simulink model "model_downsampling"  (R2021b)
settings: Solver=VariableStepAuto  StartTime=0.0  StopTime=3  RelTol=1e-3
values from neighbouring files (symbols this model uses):
  dowsampling_factor = 32    [init_model.m]
  fsample = 100e3    (= 100000)    [init_model.m]
  m1 = m1_th    [init_model.m]
  m2 = m2_th    [init_model.m]
  taps = fir1(floor(n),fpass/fsample)    [init_model.m]
  taps1 = fir1(floor(n1),fpass1/fsample)    [init_model.m]
libraries: simulink x3
settings Model: Creator=pablo  LastModifiedBy=pablo
settings SolverCC: AutoInsertRateTranBlk=on
settings DebuggingCC: SingleTaskRateTransMsg=error

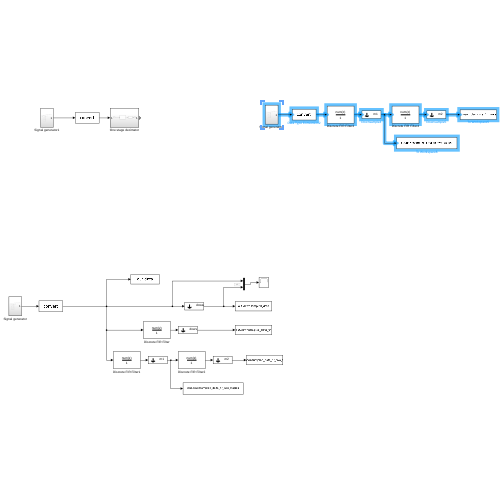
[thumbnail: Simulink's stored preview of the top-level diagram]
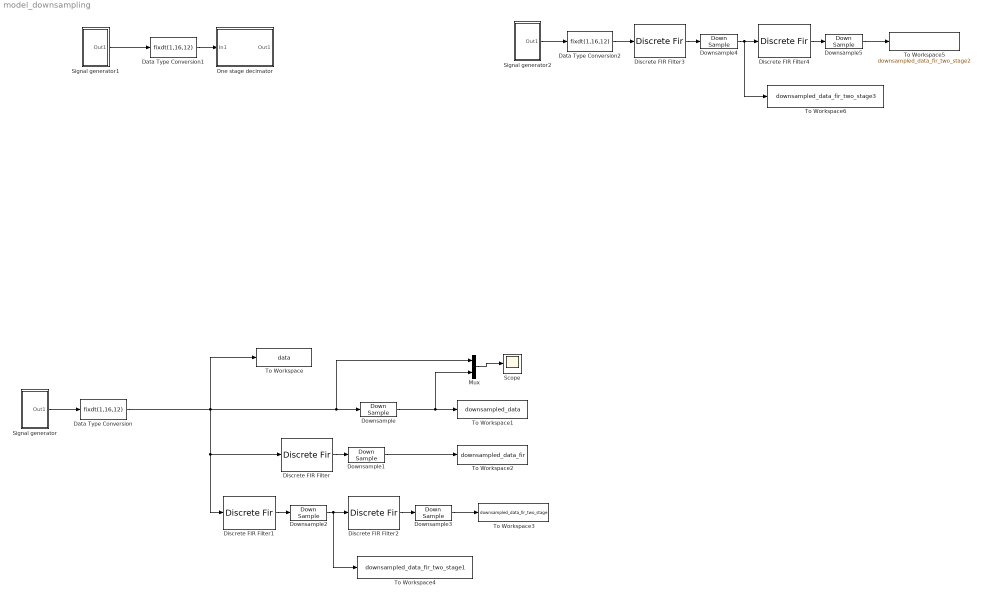
== system model_downsampling ==
  Data Type Conversion : DataTypeConversion  OutDataTypeStr=fixdt(1,16,12)
  Data Type Conversion1 : DataTypeConversion  OutDataTypeStr=fixdt(1,16,12)
  Data Type Conversion2 : DataTypeConversion  OutDataTypeStr=fixdt(1,16,12)
  Discrete FIR Filter : DiscreteFir  Coefficients=taps  InputProcessing=Columns as channels (frame based)  SampleTime=1/fsample  OutDataTypeStr=Inherit: Same as input
  Discrete FIR Filter1 : DiscreteFir  Coefficients=taps1  InputProcessing=Columns as channels (frame based)  SampleTime=1/fsample  OutDataTypeStr=Inherit: Same as input
  Discrete FIR Filter2 : DiscreteFir  Coefficients=taps1  InputProcessing=Columns as channels (frame based)  OutDataTypeStr=Inherit: Same as input
  Discrete FIR Filter3 : DiscreteFir  Coefficients=taps1  InputProcessing=Columns as channels (frame based)  SampleTime=1/fsample  OutDataTypeStr=Inherit: Same as input
  Discrete FIR Filter4 : DiscreteFir  Coefficients=taps1  InputProcessing=Columns as channels (frame based)  OutDataTypeStr=Inherit: Same as input
  Downsample : DownSample  N=dowsampling_factor  RateOptions=Allow multirate processing
  Downsample1 : DownSample  N=dowsampling_factor  RateOptions=Allow multirate processing
  Downsample2 : DownSample  N=m1  RateOptions=Allow multirate processing
  Downsample3 : DownSample  N=m2  RateOptions=Allow multirate processing
  Downsample4 : DownSample  N=m1  RateOptions=Allow multirate processing
  Downsample5 : DownSample  N=m2  RateOptions=Allow multirate processing
  Mux : Mux  Inputs=2
  One stage decimator : Subsystem
  Scope : Scope
  Signal generator : Subsystem
  Signal generator1 : Subsystem
  Signal generator2 : Subsystem
  To Workspace : ToWorkspace  VariableName=data  SampleTime=-1
  To Workspace1 : ToWorkspace  VariableName=downsampled_data  SampleTime=-1
  To Workspace2 : ToWorkspace  VariableName=downsampled_data_fir  SampleTime=-1
  To Workspace3 : ToWorkspace  VariableName=downsampled_data_fir_two_stage  SampleTime=-1
  To Workspace4 : ToWorkspace  VariableName=downsampled_data_fir_two_stage1  SampleTime=-1
  To Workspace5 : ToWorkspace  VariableName=downsampled_data_fir_two_stage2  SampleTime=-1
  To Workspace6 : ToWorkspace  VariableName=downsampled_data_fir_two_stage3  SampleTime=-1
  wires:
  Mux/1 -> Scope/1
  Downsample/1 -> To Workspace1/1, Mux/2
  Discrete FIR Filter/1 -> Downsample1/1
  Downsample1/1 -> To Workspace2/1
  Data Type Conversion/1 -> Discrete FIR Filter1/1, Discrete FIR Filter/1, Mux/1, Downsample/1, To Workspace/1
  Discrete FIR Filter1/1 -> Downsample2/1
  Discrete FIR Filter2/1 -> Downsample3/1
  Downsample2/1 -> To Workspace4/1, Discrete FIR Filter2/1
  Downsample3/1 -> To Workspace3/1
  Signal generator/1(Out1) -> Data Type Conversion/1
  Signal generator1/1(Out1) -> Data Type Conversion1/1
  Data Type Conversion1/1 -> One stage decimator/1(In1)
  Discrete FIR Filter3/1 -> Downsample4/1
  Downsample4/1 -> To Workspace6/1, Discrete FIR Filter4/1
  Downsample5/1 -> To Workspace5/1
  Discrete FIR Filter4/1 -> Downsample5/1
  Signal generator2/1(Out1) -> Data Type Conversion2/1
  Data Type Conversion2/1 -> Discrete FIR Filter3/1

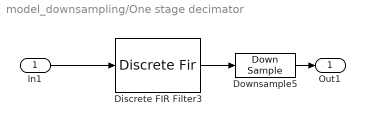
== system model_downsampling/One stage decimator ==
  In1 : Inport
  Discrete FIR Filter3 : DiscreteFir  Coefficients=taps  InputProcessing=Columns as channels (frame based)  SampleTime=1/fsample  OutDataTypeStr=Inherit: Same as input
  Downsample5 : DownSample  N=dowsampling_factor  RateOptions=Allow multirate processing
  Out1 : Outport
  wires:
  In1/1 -> Discrete FIR Filter3/1
  Downsample5/1 -> Out1/1
  Discrete FIR Filter3/1 -> Downsample5/1

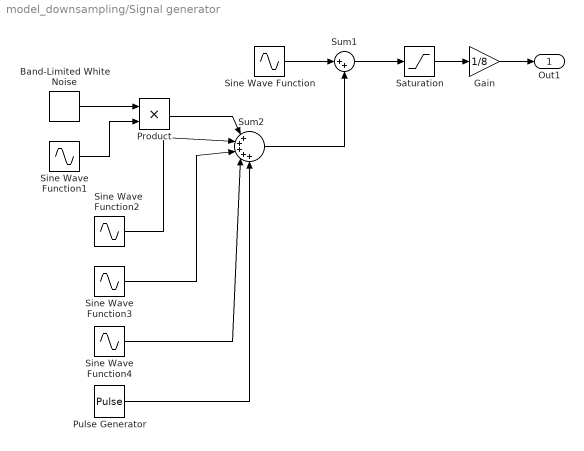
== system model_downsampling/Signal generator ==
  Band-Limited White Noise : simulink/Sources/Band-Limited White Noise  Cov=[0.00001]  Ts=1/fsample  seed=[25]
  Gain : Gain  Gain=1/8
  Product : Product
  Pulse Generator : DiscretePulseGenerator  Amplitude=0.8  Period=24  PulseWidth=12  SampleTime=1/fsample
  Saturation : Saturate  UpperLimit=8  LowerLimit=-8
  Sine Wave Function : Sin  SineType=Sample based  Frequency=50*2*pi  Samples=fsample/50  SampleTime=1/fsample
  Sine Wave Function1 : Sin  Frequency=200*2*pi  Samples=fsample/50  SampleTime=1/fsample
  Sine Wave Function2 : Sin  Amplitude=0.3  Frequency=3100*2*pi  Phase=3  Samples=fsample/50  SampleTime=1/fsample
  Sine Wave Function3 : Sin  Amplitude=0.5  Frequency=2500*2*pi  Samples=fsample/50  SampleTime=1/fsample
  Sine Wave Function4 : Sin  Amplitude=0.5  Frequency=5000*2*pi  Samples=fsample/50  SampleTime=1/fsample
  Sum1 : Sum  Inputs=|++
  Sum2 : Sum  Inputs=|+++++
  Out1 : Outport
  wires:
  Sine Wave Function2/1 -> Sum2/2
  Sine Wave Function3/1 -> Sum2/3
  Sine Wave Function/1 -> Sum1/1
  Sine Wave Function4/1 -> Sum2/4
  Sine Wave Function1/1 -> Product/2
  Band-Limited White Noise/1 -> Product/1
  Product/1 -> Sum2/1
  Pulse Generator/1 -> Sum2/5
  Sum2/1 -> Sum1/2
  Sum1/1 -> Saturation/1
  Saturation/1 -> Gain/1
  Gain/1 -> Out1/1

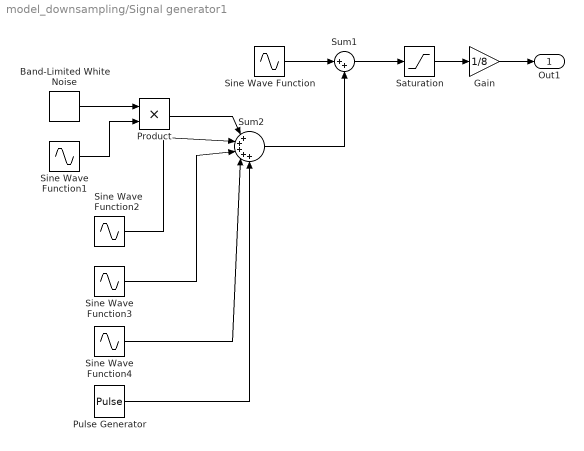
== system model_downsampling/Signal generator1 ==
  Band-Limited White Noise : simulink/Sources/Band-Limited White Noise  Cov=[0.00001]  Ts=1/fsample  seed=[25]
  Gain : Gain  Gain=1/8
  Product : Product
  Pulse Generator : DiscretePulseGenerator  Amplitude=0.8  Period=24  PulseWidth=12  SampleTime=1/fsample
  Saturation : Saturate  UpperLimit=8  LowerLimit=-8
  Sine Wave Function : Sin  SineType=Sample based  Frequency=50*2*pi  Samples=fsample/50  SampleTime=1/fsample
  Sine Wave Function1 : Sin  Frequency=200*2*pi  Samples=fsample/50  SampleTime=1/fsample
  Sine Wave Function2 : Sin  Amplitude=0.3  Frequency=3100*2*pi  Phase=3  Samples=fsample/50  SampleTime=1/fsample
  Sine Wave Function3 : Sin  Amplitude=0.5  Frequency=2500*2*pi  Samples=fsample/50  SampleTime=1/fsample
  Sine Wave Function4 : Sin  Amplitude=0.5  Frequency=5000*2*pi  Samples=fsample/50  SampleTime=1/fsample
  Sum1 : Sum  Inputs=|++
  Sum2 : Sum  Inputs=|+++++
  Out1 : Outport
  wires:
  Sine Wave Function2/1 -> Sum2/2
  Sine Wave Function3/1 -> Sum2/3
  Sine Wave Function/1 -> Sum1/1
  Sine Wave Function4/1 -> Sum2/4
  Sine Wave Function1/1 -> Product/2
  Band-Limited White Noise/1 -> Product/1
  Product/1 -> Sum2/1
  Pulse Generator/1 -> Sum2/5
  Sum2/1 -> Sum1/2
  Sum1/1 -> Saturation/1
  Saturation/1 -> Gain/1
  Gain/1 -> Out1/1

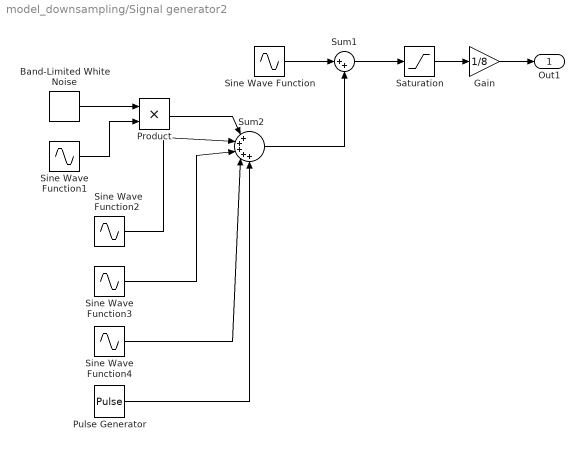
== system model_downsampling/Signal generator2 ==
  Band-Limited White Noise : simulink/Sources/Band-Limited White Noise  Cov=[0.00001]  Ts=1/fsample  seed=[25]
  Gain : Gain  Gain=1/8
  Product : Product
  Pulse Generator : DiscretePulseGenerator  Amplitude=0.8  Period=24  PulseWidth=12  SampleTime=1/fsample
  Saturation : Saturate  UpperLimit=8  LowerLimit=-8
  Sine Wave Function : Sin  SineType=Sample based  Frequency=50*2*pi  Samples=fsample/50  SampleTime=1/fsample
  Sine Wave Function1 : Sin  Frequency=200*2*pi  Samples=fsample/50  SampleTime=1/fsample
  Sine Wave Function2 : Sin  Amplitude=0.3  Frequency=3100*2*pi  Phase=3  Samples=fsample/50  SampleTime=1/fsample
  Sine Wave Function3 : Sin  Amplitude=0.5  Frequency=2500*2*pi  Samples=fsample/50  SampleTime=1/fsample
  Sine Wave Function4 : Sin  Amplitude=0.5  Frequency=5000*2*pi  Samples=fsample/50  SampleTime=1/fsample
  Sum1 : Sum  Inputs=|++
  Sum2 : Sum  Inputs=|+++++
  Out1 : Outport
  wires:
  Sine Wave Function2/1 -> Sum2/2
  Sine Wave Function3/1 -> Sum2/3
  Sine Wave Function/1 -> Sum1/1
  Sine Wave Function4/1 -> Sum2/4
  Sine Wave Function1/1 -> Product/2
  Band-Limited White Noise/1 -> Product/1
  Product/1 -> Sum2/1
  Pulse Generator/1 -> Sum2/5
  Sum2/1 -> Sum1/2
  Sum1/1 -> Saturation/1
  Saturation/1 -> Gain/1
  Gain/1 -> Out1/1
